simulink model "mvdc_KF_NonlinSingleTrack"  (R2018b)
settings: configuration reference "Active" (kept outside this file)
undefined symbols (not defined in the file): P_VDC_CovDelta_rad2, P_VDC_CovDriveForce_kN2, P_VDC_measCov_GPS, P_VDC_measCov_velocity, P_VDC_measCov_VLOC, P_VDC_OutlierBounds, P_VDC_Var_yawRate_radps, P_VDC_YawAngleDepCovMode, res_dGPS_m, res_dPsi_radps, res_dVLOC_m, res_PsiGPS_rad, res_PsiVLOC_rad, res_sGPS_m, res_sVLOC_m, res_vx_mps, res_vy_mps, res_xGPS_m, res_xVLOC_m, res_yGPS_m, res_yVLOC_m, tS, vehiclemass_kg
libraries: rr_general x2
settings Model: DataDictionary=mvdc_KF.sldd  Creator=wischnewski  LastModifiedBy=Kappertz

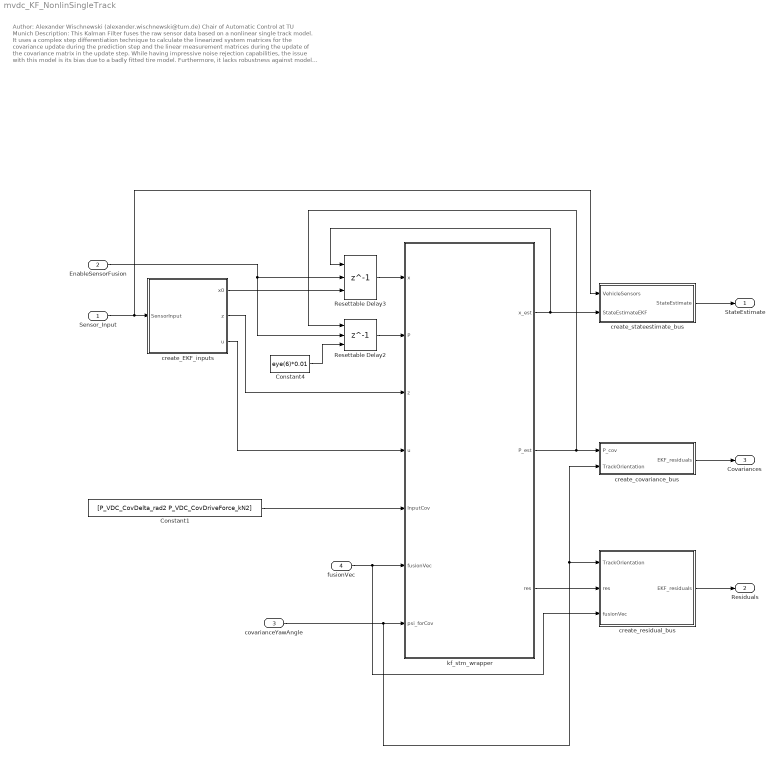
== system mvdc_KF_NonlinSingleTrack ==
  note: Author: Alexander Wischnewski (alexander.wischnewski@tum.de)
      | Chair of Automatic Control at TU Munich
      |
      | Description: This Kalman Filter fuses the raw sensor data based on a nonlinear single track model. It uses a complex step differentiation technique to
      | calculate the linearized system matrices for the covariance update during the prediction step and the linear measurement matrices during the update of the covariance matrix in the update step. While having impressive noise rejection capabilities, the issue with this model is its bias due to a badly fitted tire model. Furthermore, it lacks robustness against model errors and might become unstable.
      |
      | Inputs:
      | EnableSensorFusion Enable bit which activates the Kalman Filter
      | VehicleSensorData Raw sensor data
      | ActualPathOrientation Path orientation provided by the trajectory planner (used for weighting GPS and LIDAR via Covariance Matrix)
      | fusionVec Vector with bit-wise information about whether a sensor should be used for fusion or not
      |
      | Outputs:
      | StateEstimate Estimated state vector of the Kalman Filter
      | Residuals Pre-update measurement residuals of the Kalman Filter
      | Covariances Post-update Estimation Covariance Matrix of the Kalman Filter
  Sensor_Input : Inport  OutDataTypeStr=Bus: VehicleSensorData
  EnableSensorFusion : Inport  Port=2  OutDataTypeStr=boolean
  covarianceYawAngle : Inport  Port=3
  fusionVec : Inport  Port=4  OutDataTypeStr=boolean  PortDimensions=9
  Constant1 : Constant  Value=[P_VDC_CovDelta_rad2 P_VDC_CovDriveForce_kN2]
  Constant4 : Constant  Value=eye(6)*0.01
  Resettable Delay2 : Delay  DelayLength=1  DelayLengthUpperLimit=2  InitialConditionSource=Input port  ExternalReset=Rising
      settings: InputPortMap=u0,r5,p4
  Resettable Delay3 : Delay  DelayLength=1  DelayLengthUpperLimit=2  InitialConditionSource=Input port  ExternalReset=Rising
      settings: InputPortMap=u0,r5,p4
  create_EKF_inputs : Subsystem
  create_covariance_bus : Subsystem
  create_residual_bus : Subsystem
  create_stateestimate_bus : Subsystem
  kf_stm_wrapper : MATLAB Function  TreatAsAtomicUnit=on
  "StateEstimate " : Outport  OutDataTypeStr=Bus: StateEstimation_state
  Residuals : Outport  Port=2  OutDataTypeStr=Bus: StateEstimation_residuals
  Covariances : Outport  Port=3  OutDataTypeStr=Bus: StateEstimation_covariances
  wires:
  Sensor_Input/1 -> create_stateestimate_bus/1(VehicleSensors), create_EKF_inputs/1(SensorInput)
  kf_stm_wrapper/1(x_est) -> Resettable Delay3/1, create_stateestimate_bus/2(StateEstimateEKF)
  Resettable Delay2/1 -> kf_stm_wrapper/2(P)
  create_residual_bus/1(EKF_residuals) -> Residuals/1
  covarianceYawAngle/1 -> create_covariance_bus/2(TrackOrientation), create_residual_bus/1(TrackOrientation), kf_stm_wrapper/7(psi_forCov)
  EnableSensorFusion/1 -> Resettable Delay2/2, Resettable Delay3/2
  Resettable Delay3/1 -> kf_stm_wrapper/1(x)
  kf_stm_wrapper/2(P_est) -> Resettable Delay2/1, create_covariance_bus/1(P_cov)
  Constant4/1 -> Resettable Delay2/3
  create_covariance_bus/1(EKF_residuals) -> Covariances/1
  create_stateestimate_bus/1(StateEstimate) -> "StateEstimate "/1
  create_EKF_inputs/1(x0) -> Resettable Delay3/3
  create_EKF_inputs/2(z) -> kf_stm_wrapper/3(z)
  create_EKF_inputs/3(u) -> kf_stm_wrapper/4(u)
  Constant1/1 -> kf_stm_wrapper/5(InputCov)
  kf_stm_wrapper/3(res) -> create_residual_bus/2(res)
  fusionVec/1 -> kf_stm_wrapper/6(fusionVec), create_residual_bus/3(fusionVec)

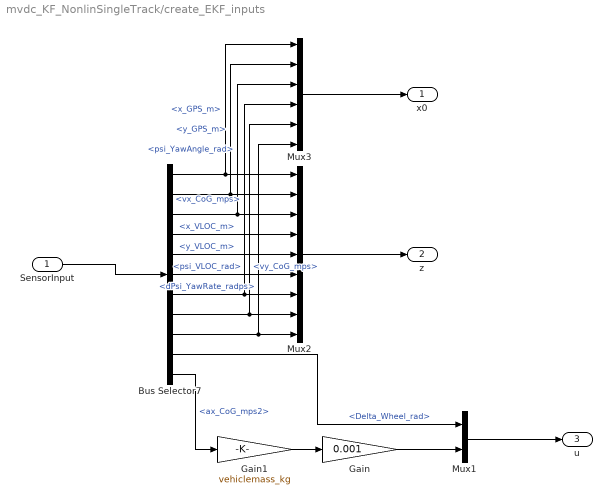
== system mvdc_KF_NonlinSingleTrack/create_EKF_inputs ==
  SensorInput : Inport
  Bus Selector7 : BusSelector  OutputSignals=x_GPS_m,y_GPS_m,psi_YawAngle_rad,x_VLOC_m,y_VLOC_m,psi_VLOC_rad,vx_CoG_mps,vy_CoG_mps,dPsi_YawRate_radps,Delta_Wheel_rad,ax_CoG_mps2
  Gain : Gain  Gain=0.001
  Gain1 : Gain  Gain=vehiclemass_kg
  Mux1 : Mux  Inputs=2
  Mux2 : Mux  Inputs=9
  Mux3 : Mux  Inputs=6
  x0 : Outport
  z : Outport  Port=2
  u : Outport  Port=3
  wires:
  SensorInput/1 -> Bus Selector7/1
  Bus Selector7/1 -> Mux3/1, Mux2/1  "<x_GPS_m>"
  Bus Selector7/2 -> Mux3/2, Mux2/2  "<y_GPS_m>"
  Mux2/1 -> z/1
  Mux3/1 -> x0/1
  Bus Selector7/5 -> Mux2/5  "<y_VLOC_m>"
  Bus Selector7/3 -> Mux3/3, Mux2/3  "<psi_YawAngle_rad>"
  Bus Selector7/9 -> Mux3/6, Mux2/9  "<dPsi_YawRate_radps>"
  Bus Selector7/7 -> Mux3/4, Mux2/7  "<vx_CoG_mps>"
  Bus Selector7/6 -> Mux2/6  "<psi_VLOC_rad>"
  Bus Selector7/4 -> Mux2/4  "<x_VLOC_m>"
  Bus Selector7/8 -> Mux3/5, Mux2/8  "<vy_CoG_mps>"
  Mux1/1 -> u/1
  Gain/1 -> Mux1/2
  Bus Selector7/10 -> Mux1/1  "<Delta_Wheel_rad>"
  Gain1/1 -> Gain/1
  Bus Selector7/11 -> Gain1/1  "<ax_CoG_mps2>"

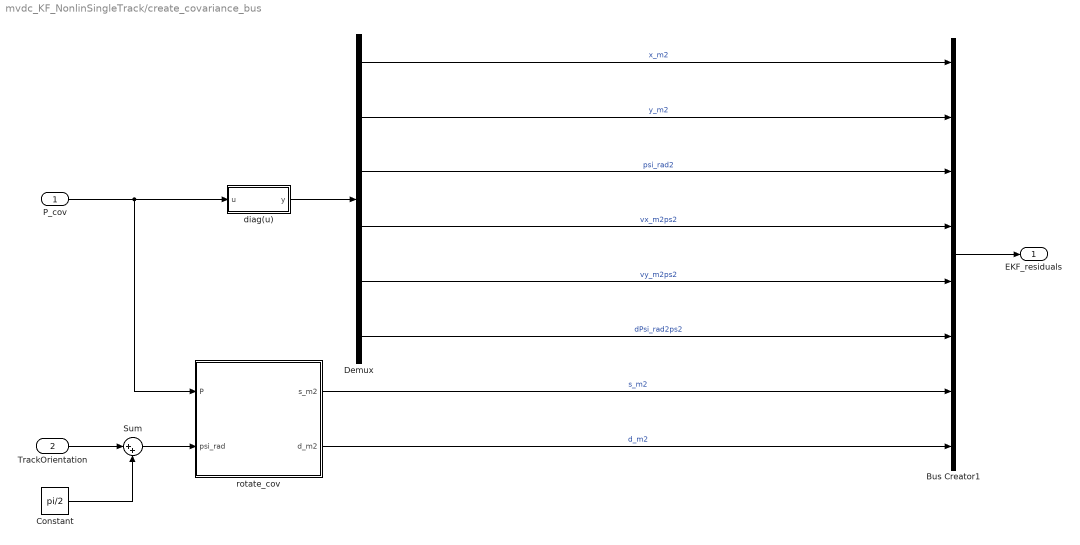
== system mvdc_KF_NonlinSingleTrack/create_covariance_bus ==
  P_cov : Inport
  TrackOrientation : Inport  Port=2
  Bus Creator1 : BusCreator  Inputs=8
  Constant : Constant  Value=pi/2
  Demux : Demux  Outputs=6
  Sum : Sum  Inputs=|++
  diag(u) : MATLAB Function  TreatAsAtomicUnit=on
  rotate_cov : MATLAB Function  TreatAsAtomicUnit=on
  EKF_residuals : Outport
  wires:
  Bus Creator1/1 -> EKF_residuals/1
  TrackOrientation/1 -> Sum/1
  Constant/1 -> Sum/2
  P_cov/1 -> diag(u)/1(u), rotate_cov/1(P)
  diag(u)/1(y) -> Demux/1
  Demux/1 -> Bus Creator1/1  "x_m2"
  Demux/2 -> Bus Creator1/2  "y_m2"
  Demux/3 -> Bus Creator1/3  "psi_rad2"
  Demux/4 -> Bus Creator1/4  "vx_m2ps2"
  Demux/5 -> Bus Creator1/5  "vy_m2ps2"
  Demux/6 -> Bus Creator1/6  "dPsi_rad2ps2"
  rotate_cov/1(s_m2) -> Bus Creator1/7  "s_m2"
  rotate_cov/2(d_m2) -> Bus Creator1/8  "d_m2"
  Sum/1 -> rotate_cov/2(psi_rad)

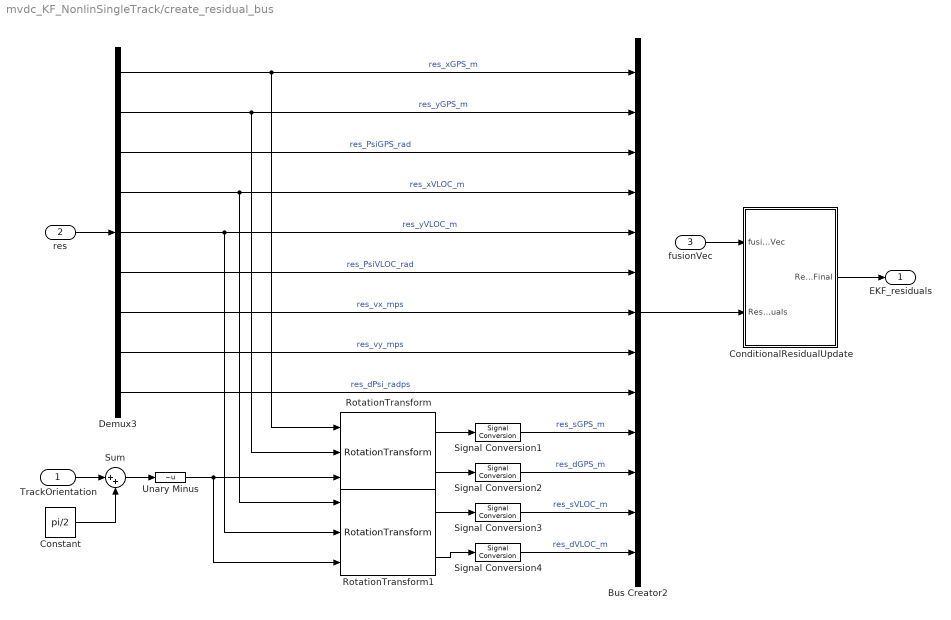
== system mvdc_KF_NonlinSingleTrack/create_residual_bus ==
  TrackOrientation : Inport
  res : Inport  Port=2
  fusionVec : Inport  Port=3
  Bus Creator2 : BusCreator  Inputs=13
  ConditionalResidualUpdate : Subsystem
  Constant : Constant  Value=pi/2
  Demux3 : Demux  Outputs=9
  RotationTransform : rr_general/RotationTransform  SystemSampleTime=-1
  RotationTransform1 : rr_general/RotationTransform  SystemSampleTime=-1
  Signal Conversion{1..4} (4 alike) : SignalConversion  OverrideOpt=off
  Sum : Sum  Inputs=|++
  Unary Minus : UnaryMinus
  EKF_residuals : Outport
  wires:
  Demux3/3 -> Bus Creator2/3  "res_PsiGPS_rad"
  Demux3/1 -> RotationTransform/1, Bus Creator2/1  "res_xGPS_m"
  Demux3/2 -> RotationTransform/2, Bus Creator2/2  "res_yGPS_m"
  RotationTransform/1 -> Signal Conversion1/1
  RotationTransform/2 -> Signal Conversion2/1
  RotationTransform1/2 -> Signal Conversion4/1
  RotationTransform1/1 -> Signal Conversion3/1
  Unary Minus/1 -> RotationTransform1/3, RotationTransform/3
  TrackOrientation/1 -> Sum/1
  Constant/1 -> Sum/2
  Sum/1 -> Unary Minus/1
  Signal Conversion1/1 -> Bus Creator2/10  "res_sGPS_m"
  Signal Conversion2/1 -> Bus Creator2/11  "res_dGPS_m"
  Signal Conversion3/1 -> Bus Creator2/12  "res_sVLOC_m"
  Signal Conversion4/1 -> Bus Creator2/13  "res_dVLOC_m"
  fusionVec/1 -> ConditionalResidualUpdate/1(fusionVec)
  res/1 -> Demux3/1
  Bus Creator2/1 -> ConditionalResidualUpdate/2(Residuals)
  ConditionalResidualUpdate/1(ResidualsFinal) -> EKF_residuals/1
  Demux3/4 -> RotationTransform1/1, Bus Creator2/4  "res_xVLOC_m"
  Demux3/5 -> RotationTransform1/2, Bus Creator2/5  "res_yVLOC_m"
  Demux3/6 -> Bus Creator2/6  "res_PsiVLOC_rad"
  Demux3/7 -> Bus Creator2/7  "res_vx_mps"
  Demux3/8 -> Bus Creator2/8  "res_vy_mps"
  Demux3/9 -> Bus Creator2/9  "res_dPsi_radps"

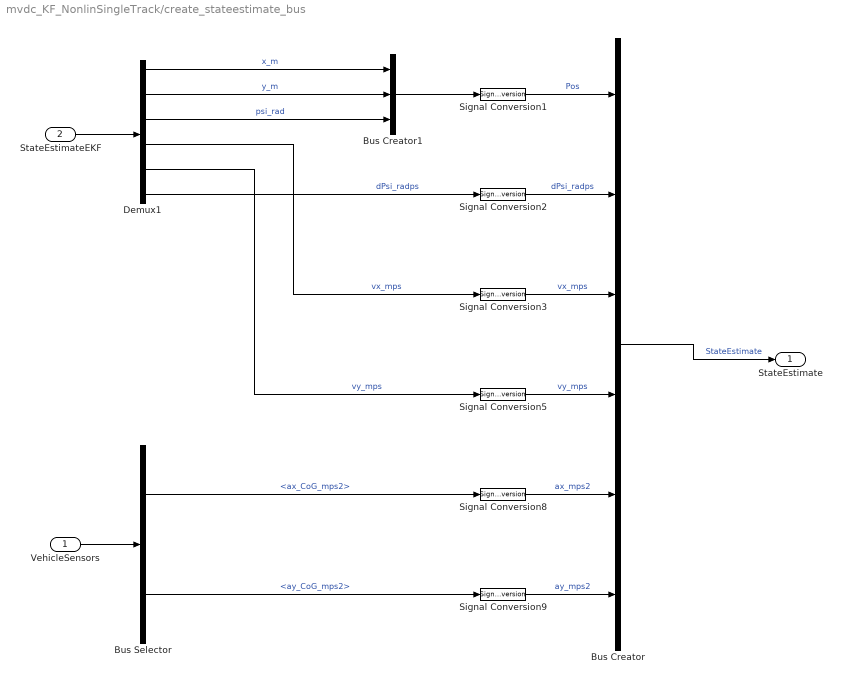
== system mvdc_KF_NonlinSingleTrack/create_stateestimate_bus ==
  VehicleSensors : Inport
  StateEstimateEKF : Inport  Port=2
  Bus Creator : BusCreator  Inputs=6
  Bus Creator1 : BusCreator  Inputs=3  OutDataTypeStr=Bus: CartPos
  Bus Selector : BusSelector  OutputSignals=ax_CoG_mps2,ay_CoG_mps2
  Demux1 : Demux  Outputs=6
  Signal Conversion{1..3,5,8..9} (6 alike) : SignalConversion  OverrideOpt=off
  StateEstimate : Outport
  wires:
  StateEstimateEKF/1 -> Demux1/1
  Signal Conversion2/1 -> Bus Creator/2  "dPsi_radps"
  Signal Conversion9/1 -> Bus Creator/6  "ay_mps2"
  Bus Selector/2 -> Signal Conversion9/1  "<ay_CoG_mps2>"
  Bus Creator/1 -> StateEstimate/1  "StateEstimate"
  Demux1/4 -> Signal Conversion3/1  "vx_mps"
  Bus Selector/1 -> Signal Conversion8/1  "<ax_CoG_mps2>"
  Signal Conversion5/1 -> Bus Creator/4  "vy_mps"
  Signal Conversion3/1 -> Bus Creator/3  "vx_mps"
  Signal Conversion8/1 -> Bus Creator/5  "ax_mps2"
  Demux1/5 -> Signal Conversion5/1  "vy_mps"
  Demux1/3 -> Bus Creator1/3  "psi_rad"
  Demux1/6 -> Signal Conversion2/1  "dPsi_radps"
  Bus Creator1/1 -> Signal Conversion1/1
  Signal Conversion1/1 -> Bus Creator/1  "Pos"
  Demux1/1 -> Bus Creator1/1  "x_m"
  Demux1/2 -> Bus Creator1/2  "y_m"
  VehicleSensors/1 -> Bus Selector/1

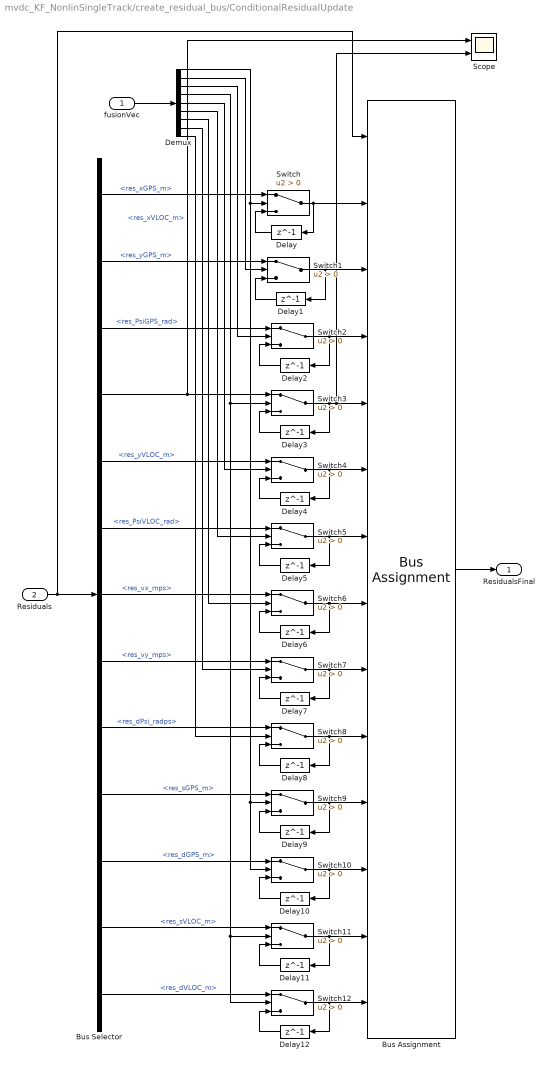
== system mvdc_KF_NonlinSingleTrack/create_residual_bus/ConditionalResidualUpdate ==
  fusionVec : Inport
  Residuals : Inport  Port=2
  Bus Assignment : BusAssignment  AssignedSignals=res_xGPS_m,res_yGPS_m,res_PsiGPS_rad,res_xVLOC_m,res_yVLOC_m,res_PsiVLOC_rad,res_vx_mps,res_vy_mps,res_dPsi_radps,res_sGPS_m,res_dGPS_m,res_sVLOC_m,res_dVLOC_m
  Bus Selector : BusSelector  OutputSignals=res_xGPS_m,res_yGPS_m,res_PsiGPS_rad,res_xVLOC_m,res_yVLOC_m,res_PsiVLOC_rad,res_vx_mps,res_vy_mps,res_dPsi_radps,res_sGPS_m,res_dGPS_m,res_sVLOC_m,res_dVLOC_m
  Delay{,1..12} (13 alike) : Delay  DelayLength=1  InitialCondition=0
  Demux : Demux  Outputs=9
  Scope : Scope  NumInputPorts=2
  Switch{,1..12} (13 alike) : Switch  Criteria=u2 > Threshold
  ResidualsFinal : Outport
  wires:
  Demux/5 -> Switch4/2
  Delay8/1 -> Switch8/3
  Switch8/1 -> Bus Assignment/10, Delay8/1
  Bus Selector/6 -> Switch5/1  "<res_PsiVLOC_rad>"
  Switch6/1 -> Bus Assignment/8, Delay6/1
  Delay6/1 -> Switch6/3
  Demux/7 -> Switch6/2
  Switch7/1 -> Bus Assignment/9, Delay7/1
  Delay7/1 -> Switch7/3
  Switch2/1 -> Bus Assignment/4, Delay2/1
  Switch4/1 -> Bus Assignment/6, Delay4/1
  Delay4/1 -> Switch4/3
  Delay/1 -> Switch/3
  Switch/1 -> Bus Assignment/2, Delay/1
  Bus Assignment/1 -> ResidualsFinal/1
  Demux/3 -> Switch2/2
  Residuals/1 -> Bus Assignment/1, Bus Selector/1
  Bus Selector/1 -> Switch/1  "<res_xGPS_m>"
  Demux/8 -> Switch7/2
  Demux/9 -> Switch8/2
  Delay5/1 -> Switch5/3
  Switch5/1 -> Bus Assignment/7, Delay5/1
  Demux/2 -> Switch1/2
  Demux/6 -> Switch5/2
  Demux/4 -> Switch12/2, Switch11/2, Switch3/2
  Bus Selector/8 -> Switch7/1  "<res_vy_mps>"
  Delay2/1 -> Switch2/3
  Bus Selector/7 -> Switch6/1  "<res_vx_mps>"
  Delay1/1 -> Switch1/3
  Bus Selector/2 -> Switch1/1  "<res_yGPS_m>"
  Switch1/1 -> Bus Assignment/3, Delay1/1
  fusionVec/1 -> Demux/1
  Delay3/1 -> Switch3/3
  Bus Selector/9 -> Switch8/1  "<res_dPsi_radps>"
  Switch12/1 -> Bus Assignment/14, Delay12/1
  Switch10/1 -> Bus Assignment/12, Delay10/1
  Switch11/1 -> Bus Assignment/13, Delay11/1
  Switch9/1 -> Bus Assignment/11, Delay9/1
  Bus Selector/10 -> Switch9/1  "<res_sGPS_m>"
  Delay9/1 -> Switch9/3
  Delay10/1 -> Switch10/3
  Delay11/1 -> Switch11/3
  Delay12/1 -> Switch12/3
  Bus Selector/13 -> Switch12/1  "<res_dVLOC_m>"
  Bus Selector/12 -> Switch11/1  "<res_sVLOC_m>"
  Bus Selector/11 -> Switch10/1  "<res_dGPS_m>"
  Demux/1 -> Switch/2, Switch10/2, Switch9/2
  Bus Selector/3 -> Switch2/1  "<res_PsiGPS_rad>"
  Bus Selector/4 -> Scope/1, Switch3/1  "<res_xVLOC_m>"
  Bus Selector/5 -> Switch4/1  "<res_yVLOC_m>"
  Switch3/1 -> Scope/2, Bus Assignment/5, Delay3/1

== matlab function mvdc_KF_NonlinSingleTrack/kf_stm_wrapper ==
  data: x input; P input; z input; u input; x_est output; P_est output; tS parameter; InputCov input; res output size=9; fusionVec input; psi_forCov input; P_VDC_Var_yawRate_radps parameter; P_VDC_measCov_VLOC parameter; P_VDC_measCov_velocity parameter; P_VDC_measCov_GPS parameter; P_VDC_OutlierBounds parameter; P_VDC_YawAngleDepCovMode parameter
function [x_est, P_est, res] = kf_stm_wrapper(x, P, z, u, tS, InputCov, fusionVec, psi_forCov, P_VDC_Var_yawRate_radps, P_VDC_measCov_VLOC, P_VDC_measCov_velocity, P_VDC_measCov_GPS, P_VDC_OutlierBounds, P_VDC_YawAngleDepCovMode)

[x_est, P_est, res]= kf_stm(x, z, u, tS, InputCov, P, P_VDC_YawAngleDepCovMode, P_VDC_OutlierBounds, fusionVec, psi_forCov, P_VDC_measCov_GPS, P_VDC_measCov_VLOC, P_VDC_measCov_velocity, P_VDC_Var_yawRate_radps);

end

== matlab function mvdc_KF_NonlinSingleTrack/create_covariance_bus/diag(u) ==
  data: u input; y output
function y = diag(u)

y=diag(u);

% end

== matlab function mvdc_KF_NonlinSingleTrack/create_covariance_bus/rotate_cov ==
  data: P input; s_m2 output; psi_rad input; d_m2 output
function [s_m2, d_m2] = rotateCov(P, psi_rad)

% construct rotation matrix
R = [cos(psi_rad), -sin(psi_rad);...
  sin(psi_rad), cos(psi_rad)];

Prot = R*P(1:2, 1:2)*R';
Prot_diag = diag(Prot); 

s_m2 = Prot_diag(1); 
d_m2 = Prot_diag(2); 

% end
